simulink model "inbuilt_functions"  (R2021a)
settings: Solver=VariableStepAuto  StartTime=0.0  StopTime=10.0  RelTol=1e-3
settings Model: Creator=Acer  LastModifiedBy=Acer

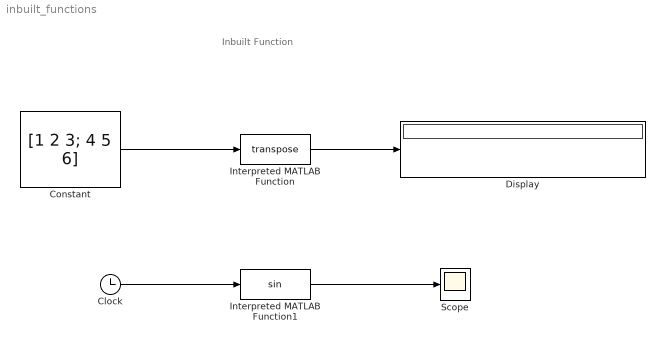
== system inbuilt_functions ==
  note: Inbuilt Function
  Clock : Clock
  Constant : Constant  Value=[1 2 3; 4 5 6]
  Display : Display
  Interpreted MATLAB Function : MATLABFcn  MATLABFcn=transpose  Output1D=off
  Interpreted MATLAB Function1 : MATLABFcn  Output1D=off
  Scope : Scope
  wires:
  Interpreted MATLAB Function/1 -> Display/1
  Constant/1 -> Interpreted MATLAB Function/1
  Interpreted MATLAB Function1/1 -> Scope/1
  Clock/1 -> Interpreted MATLAB Function1/1
